simulink model "cruise_simulink"  (R2018b)
settings: Solver=VariableStepAuto  StartTime=0.0  StopTime=10.0  RelTol=1e-3
settings Model: Creator=lobo  LastModifiedBy=lobo

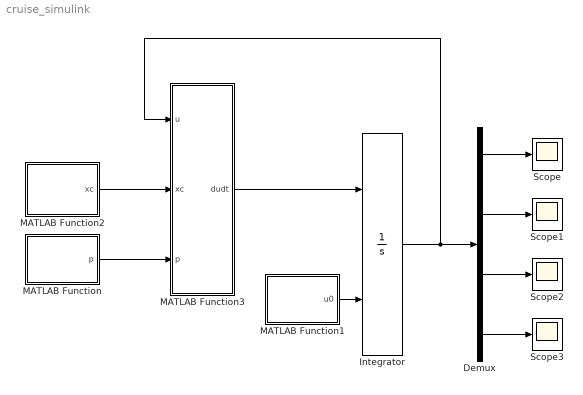
== system cruise_simulink ==
  Demux : Demux
  Integrator : Integrator  InitialConditionSource=external
  MATLAB Function : MATLAB Function  TreatAsAtomicUnit=on
  MATLAB Function1 : MATLAB Function  TreatAsAtomicUnit=on
  MATLAB Function2 : MATLAB Function  TreatAsAtomicUnit=on
  MATLAB Function3 : MATLAB Function  TreatAsAtomicUnit=on
  Scope{,1..3} (4 alike) : Scope
  wires:
  MATLAB Function/1(p) -> MATLAB Function3/3(p)
  MATLAB Function3/1(dudt) -> Integrator/1
  MATLAB Function1/1(u0) -> Integrator/2
  MATLAB Function2/1(xc) -> MATLAB Function3/2(xc)
  Integrator/1 -> MATLAB Function3/1(u), Demux/1
  Demux/1 -> Scope/1
  Demux/2 -> Scope1/1
  Demux/3 -> Scope2/1
  Demux/4 -> Scope3/1

== matlab function cruise_simulink/MATLAB Function1 ==
  data: u0 output
function u0 = IC
%{

	The following function returns the different initial conditions
    of the statement
%}

%% Initial conditions and state vector
x0 = 0; % Position
h0 = 10000; % Height
W0 = p(8); %Weight
v0 = 1.2 * (2 * p(8) / (ISA(h0) * p(2))) ^ 0.5 * (p(9) / p(5)) ^ 0.25; % Initial base velcocity

u0 = [v0, x0, h0, W0]; %Initial state vector

end

== matlab function cruise_simulink/MATLAB Function ==
  data: p output
function p = parameters
%{

	The following function returns the different parameters given in the
	statement of the problem:

	Inputs
	------
	None

	Returns
	-------
	p: array
		Array that contains all the different parameters
%}

p = zeros(10,1);

p(1)  = 47.574;                % Wingspan                       [m]
p(2)  = 286.15;                % Surface                        [m^2]
p(3)  = 7.9;                   % Aspect ratio                   [-]
p(4)  = 0.8;                   % Oswald efficiency              [-]
p(5)  = 0.018;                 % Zero-lift drag coefficient     [-]
p(6)  = 444822;                % Maximum thrust at sea level    [N]
p(7)  = 0.000167;              % Specific fuel consumption      [s^-1]
p(8)  = 1.333*10^6;            % Maximum takeoff weight         [N]
p(9)  = 1/(p(4)*pi*p(3));      % Induced drag coefficient       [-]
p(10) = 1/(2*sqrt(p(9)*p(5))); % Maximum aerodynamic efficiency [-]

end

== matlab function cruise_simulink/MATLAB Function2 ==
  data: xc output
function xc = Fun_Control()
%% INPUTS
% flag  --> Flag for the type of manoeuvre
%       --> 0 Cruise
%       --> 1 Vertical with constant elevation angle
%       --> 2 Vertical with constant thrust level
%       --> 3 Turning
% u     --> State vector
% p     --> Aircraft parameters (see Parameters.m)
%% OUTPUTS
% xc    --> Control vector (thrust level or elevation angle)
%% MAIN
xc = 1.0

end

== matlab function cruise_simulink/MATLAB Function3 ==
  data: dudt output; u input; xc input; p input
function dudt = ODE_Cruise(u,xc, p)
%% INPUTS
% t    -->  Time
% u    -->  State vector 
% u(1) -->  V (velocity)   [m/s]
% u(2) -->  x (Position)   [m]
% u(3) -->  h (Height)     [m]   
% u(4) -->  W (Weight)     [N]
% xc   -->  Thrust level   [-]
%% OUTPUTS
% dudt -->  Time derivative of u
%% MAIN
global p
g = 9.81; 

% Retrieve parameters
S = p(2);
CD0 = p(5);
k = p(9);
TmaxSL = p(6);
SFCT = p(7);

% Get state related variables
rhoSL = ISA(0);
rho = ISA(u(3));
T = xc*TmaxSL*(rho/rhoSL)^0.7;
CL = u(4)/(1/2*rho*u(1)^2*S);
D = 1/2*rho*u(1)^2*S*(CD0+k*CL^2);
W = u(4);
V = u(1);

% Get the time derivatives
dudt = zeros(4,1);
dudt(1) = (T-D)*g/W;
dudt(2) = V;
dudt(3) = 0;
dudt(4) = -SFCT*T;


end
